simulink model "complete_fusion_syste"  (R2022b)
settings: Solver=VariableStepAuto  StartTime=0.0  StopTime=45  FixedStep=t  RelTol=1e-3
values from neighbouring files (symbols this model uses):
  covA = 610    [fusion.m]    (also in fusion_parameters.m = 800; fusion_test.m = 0.00171675)
  covG = 0.76e-5    (= 7.6e-06)    [fusion.m]    (also in fusion_parameters.m = 0.0001; fusion_test.m = 0.004)
  covM = 0.4    [fusion.m]    (also in fusion_parameters.m = 80; fusion_test.m = 0)
  covP = 4    [fusion.m]    (also in fusion_parameters.m = 34; fusion_test.m = 0)
  covV = 0.01    [fusion.m]    (also in fusion_parameters.m = 0.0464; fusion_test.m = 0)
  fusion_t = 0.005    [fusion_parameters.m]
  gps_hz = 1/25    (= 0.04)    [fusion_parameters.m]
  imu_hz = 0.015    [fusion_parameters.m]
  IMUNED2VNED = rotmat(quaternion(IMU_ANGLE,"eulerd","XYZ","frame"),"frame")    [fusion_parameters.m]
  initstate = zeros(28,1)    [fusion_parameters.m]    (also in fusion_test.m)
  MAGNED2VNED = rotmat(quaternion(MAG_ANGLE,"eulerd","XYZ","frame"),"frame")    [fusion_parameters.m]
  ref_location = [40.437675, -86.943750, 680]    [fusion_parameters.m]
libraries: simulink x2, sensorgpslib x1, mspsensorlib x1
settings Model: Creator=fullb  LastModifiedBy=Inver

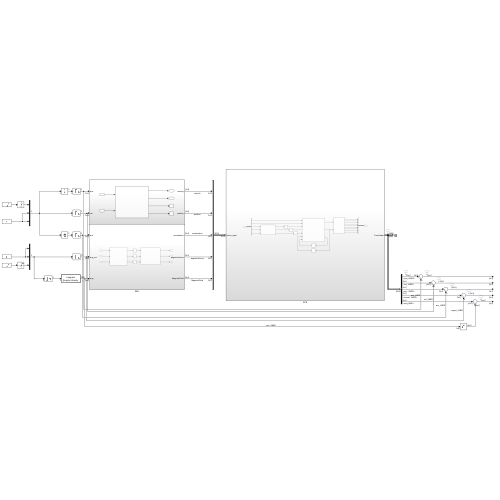
[thumbnail: Simulink's stored preview of the top-level diagram]
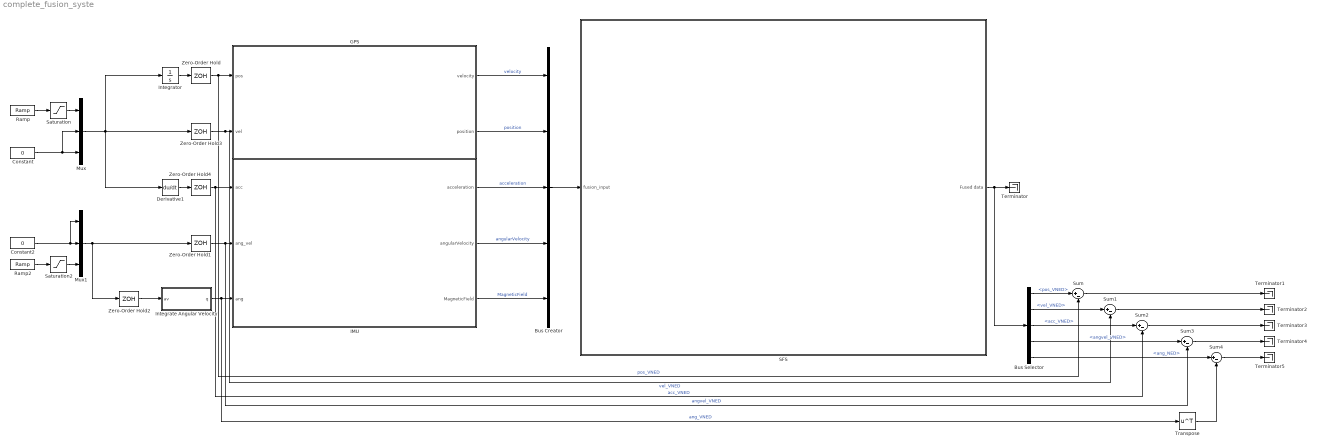
== system complete_fusion_syste ==
  Bus Creator : BusCreator  Inputs=5
  Bus Selector : BusSelector  OutputSignals=pos_VNED,vel_VNED,acc_VNED,angvel_VNED,ang_NED
  Constant : Constant  Value=0
  Constant2 : Constant  Value=0
  Derivative1 : Derivative
  GPS : Subsystem
  IMU : Subsystem
  Integrate Angular Velocity : MATLAB Function  TreatAsAtomicUnit=on  mask{rate=imu_hz}
      mask prompts: rate "Sample Rate"
  Integrator : Integrator
  Mux : Mux  Inputs=3
  Mux1 : Mux  Inputs=3
  Ramp : simulink/Sources/Ramp  slope=3  start=0  InitialOutput=-30
  Ramp2 : simulink/Sources/Ramp  slope=1  start=0  InitialOutput=-20
  SFS : Subsystem
  Saturation : Saturate  UpperLimit=10  LowerLimit=0
  Saturation2 : Saturate  UpperLimit=2  LowerLimit=0
  Sum{,1..4} (5 alike) : Sum  Inputs=|+-
  Terminator{,1..5} (6 alike) : Terminator
  Transpose : Math  Operator=transpose
  Zero-Order Hold : ZeroOrderHold  SampleTime=gps_hz
  Zero-Order Hold1 : ZeroOrderHold  SampleTime=imu_hz
  Zero-Order Hold2 : ZeroOrderHold  SampleTime=imu_hz
  Zero-Order Hold3 : ZeroOrderHold  SampleTime=gps_hz
  Zero-Order Hold4 : ZeroOrderHold  SampleTime=imu_hz
  wires:
  Bus Creator/1 -> SFS/1(fusion_input)
  SFS/1(Fused data) -> Bus Selector/1, Terminator/1
  GPS/1(velocity) -> Bus Creator/1  "velocity"
  GPS/2(position) -> Bus Creator/2  "position"
  IMU/1(acceleration) -> Bus Creator/3  "acceleration"
  IMU/2(angularVelocity) -> Bus Creator/4  "angularVelocity"
  IMU/3(MagneticField) -> Bus Creator/5  "MagneticField"
  Mux/1 -> Zero-Order Hold3/1, Derivative1/1, Integrator/1
  Derivative1/1 -> Zero-Order Hold4/1
  Ramp/1 -> Saturation/1
  Constant/1 -> Mux/2, Mux/3
  Zero-Order Hold1/1 -> Sum3/2, IMU/2(ang_vel)  "angvel_VNED"
  Zero-Order Hold2/1 -> Integrate Angular Velocity/1(av)
  Zero-Order Hold/1 -> Sum/2, GPS/1(pos)  "pos_VNED"
  Zero-Order Hold3/1 -> Sum1/2, GPS/2(vel)  "vel_VNED"
  Zero-Order Hold4/1 -> Sum2/2, IMU/1(acc)  "acc_VNED"
  Integrator/1 -> Zero-Order Hold/1
  Saturation/1 -> Mux/1
  Constant2/1 -> Mux1/1, Mux1/2
  Saturation2/1 -> Mux1/3
  Ramp2/1 -> Saturation2/1
  Mux1/1 -> Zero-Order Hold2/1, Zero-Order Hold1/1
  Integrate Angular Velocity/1(q) -> Transpose/1, IMU/3(ang)  "ang_VNED"
  Bus Selector/1 -> Sum/1  "<pos_VNED>"
  Bus Selector/2 -> Sum1/1  "<vel_VNED>"
  Bus Selector/3 -> Sum2/1  "<acc_VNED>"
  Bus Selector/4 -> Sum3/1  "<angvel_VNED>"
  Bus Selector/5 -> Sum4/1  "<ang_NED>"
  Sum/1 -> Terminator1/1
  Sum1/1 -> Terminator2/1
  Sum2/1 -> Terminator3/1
  Sum3/1 -> Terminator4/1
  Sum4/1 -> Terminator5/1
  Transpose/1 -> Sum4/2

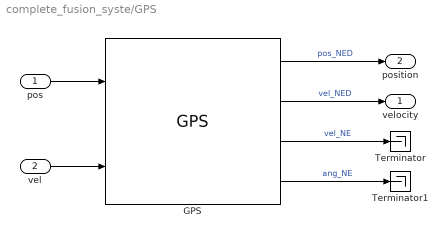
== system complete_fusion_syste/GPS ==
  pos : Inport  PortDimensions=[1 3]
  vel : Inport  Port=2  PortDimensions=[1 3]
  GPS : sensorgpslib/GPS  DispRefFrame=NED  PositionInputFormat=Local  ReferenceLocation=ref_location  HorizontalPositionAccuracy=GPS_Z_ACCURACY  VerticalPositionAccuracy=GPS_XY_ACCURACY  VelocityAccuracy=GPS_V_ACCURACY  DecayFactor=GPS_NOISE_FACTOR  SeedDouble=r_GPS  SimulateUsing=Interpreted execution
      settings: LibrarySourceBlock=mspsensorlib/GPS
  Terminator : Terminator
  Terminator1 : Terminator
  velocity : Outport
  position : Outport  Port=2
  wires:
  GPS/1 -> position/1  "pos_NED"
  GPS/2 -> velocity/1  "vel_NED"
  GPS/3 -> Terminator/1  "vel_NE"
  GPS/4 -> Terminator1/1  "ang_NE"
  pos/1 -> GPS/1
  vel/1 -> GPS/2

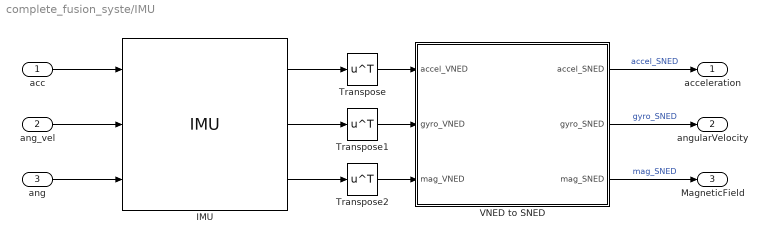
== system complete_fusion_syste/IMU ==
  acc : Inport  PortDimensions=[1 3]
  ang_vel : Inport  Port=2  PortDimensions=[1 3]
  ang : Inport  Port=3  PortDimensions=[1 4]
  IMU : mspsensorlib/IMU  DispRefFrame=NED  Temperature=25  MagneticFieldNED=ref_mag_field  MagneticFieldENU=[ -2.4169, 27.5550, 16.0849 ]  SeedDouble=r_IMU  SimulateUsing=Interpreted execution  AccelParamsMeasurementRange=ACC_MAX  AccelParamsResolution=ACC_RES  AccelParamsConstantBias=ACC_BIAS  AccelParamsAxesMisalignment=ACC_SKEW  AccelParamsNoiseDensity=ACC_VEL_WALK  AccelParamsBiasInstability=ACC_BIAS_INSTABILITY  AccelParamsRandomWalk=ACC_WALK  AccelParamsTemperatureBias=ACC_T_BIAS  AccelParamsTemperatureScaleFactor=ACC_T_SCALE  GyroParamsMeasurementRange=GYR_MAX  GyroParamsResolution=GYR_RES  GyroParamsConstantBias=GYR_BIAS  GyroParamsAxesMisalignment=GYR_SKEW  GyroParamsAccelerationBias=GYR_ACC_BIAS  GyroParamsNoiseDensity=GYR_ANG_WALK  GyroParamsBiasInstability=GYR_BIAS_INSTABILITY  GyroParamsRandomWalk=GYR_WALK  GyroParamsTemperatureBias=GYR_T_BIAS  GyroParamsTemperatureScaleFactor=GYR_T_SCALE  MagParamsMeasurementRange=MAG_MAX  MagParamsResolution=MAG_RES  MagParamsConstantBias=MAG_BIAS  MagParamsAxesMisalignment=MAG_SKEW  MagParamsNoiseDensity=MAG_WHITE  MagParamsBiasInstability=MAG_BIAS_INSTABILITY  MagParamsRandomWalk=MAG_WALK  MagParamsTemperatureBias=MAG_T_BIAS  MagParamsTemperatureScaleFactor=MAG_T_SCALE
  Transpose : Math  Operator=transpose
  Transpose1 : Math  Operator=transpose
  Transpose2 : Math  Operator=transpose
  VNED to SNED : MATLAB Function  TreatAsAtomicUnit=on
  acceleration : Outport
  angularVelocity : Outport  Port=2
  MagneticField : Outport  Port=3
  wires:
  IMU/1 -> Transpose/1
  IMU/2 -> Transpose1/1
  IMU/3 -> Transpose2/1
  ang_vel/1 -> IMU/2
  ang/1 -> IMU/3
  acc/1 -> IMU/1
  VNED to SNED/3(mag_SNED) -> MagneticField/1  "mag_SNED"
  VNED to SNED/2(gyro_SNED) -> angularVelocity/1  "gyro_SNED"
  VNED to SNED/1(accel_SNED) -> acceleration/1  "accel_SNED"
  Transpose/1 -> VNED to SNED/1(accel_VNED)
  Transpose1/1 -> VNED to SNED/2(gyro_VNED)
  Transpose2/1 -> VNED to SNED/3(mag_VNED)

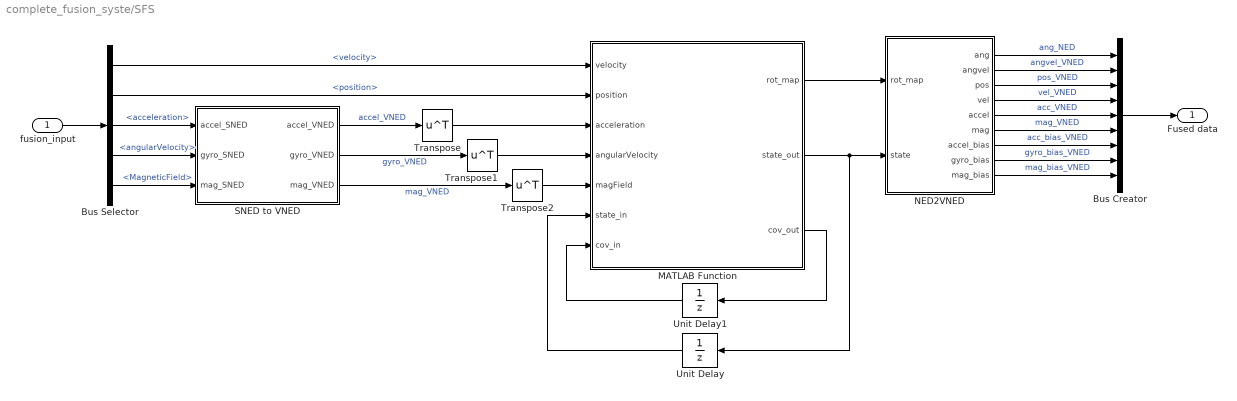
== system complete_fusion_syste/SFS ==
  fusion_input : Inport
  Bus Creator : BusCreator  Inputs=9
  Bus Selector : BusSelector  OutputSignals=velocity,position,acceleration,angularVelocity,MagneticField
  MATLAB Function : MATLAB Function  TreatAsAtomicUnit=on  SystemSampleTime=fusion_t
  NED2VNED : MATLAB Function  TreatAsAtomicUnit=on
  SNED to VNED : MATLAB Function  TreatAsAtomicUnit=on  SystemSampleTime=fusion_t
  Transpose : Math  Operator=transpose
  Transpose1 : Math  Operator=transpose
  Transpose2 : Math  Operator=transpose
  Unit Delay : UnitDelay  InitialCondition=initstate  SampleTime=fusion_t  HasFrameUpgradeWarning=on
  Unit Delay1 : UnitDelay  InitialCondition=eye(28)./1000  SampleTime=fusion_t  HasFrameUpgradeWarning=on
  Fused data : Outport
  wires:
  Bus Selector/1 -> MATLAB Function/1(velocity)  "<velocity>"
  Bus Selector/4 -> SNED to VNED/2(gyro_SNED)  "<angularVelocity>"
  Unit Delay/1 -> MATLAB Function/6(state_in)
  MATLAB Function/2(state_out) -> Unit Delay/1, NED2VNED/2(state)
  Bus Selector/2 -> MATLAB Function/2(position)  "<position>"
  Bus Selector/3 -> SNED to VNED/1(accel_SNED)  "<acceleration>"
  fusion_input/1 -> Bus Selector/1
  Bus Selector/5 -> SNED to VNED/3(mag_SNED)  "<MagneticField>"
  MATLAB Function/1(rot_map) -> NED2VNED/1(rot_map)
  Bus Creator/1 -> Fused data/1
  SNED to VNED/2(gyro_VNED) -> Transpose1/1  "gyro_VNED"
  SNED to VNED/1(accel_VNED) -> Transpose/1  "accel_VNED"
  SNED to VNED/3(mag_VNED) -> Transpose2/1  "mag_VNED"
  MATLAB Function/3(cov_out) -> Unit Delay1/1
  Unit Delay1/1 -> MATLAB Function/7(cov_in)
  NED2VNED/1(ang) -> Bus Creator/1  "ang_NED"
  NED2VNED/2(angvel) -> Bus Creator/2  "angvel_VNED"
  NED2VNED/6(mag) -> Bus Creator/6  "mag_VNED"
  NED2VNED/3(pos) -> Bus Creator/3  "pos_VNED"
  NED2VNED/4(vel) -> Bus Creator/4  "vel_VNED"
  NED2VNED/5(accel) -> Bus Creator/5  "acc_VNED"
  NED2VNED/7(accel_bias) -> Bus Creator/7  "acc_bias_VNED"
  NED2VNED/8(gyro_bias) -> Bus Creator/8  "gyro_bias_VNED"
  NED2VNED/9(mag_bias) -> Bus Creator/9  "mag_bias_VNED"
  Transpose/1 -> MATLAB Function/3(acceleration)
  Transpose1/1 -> MATLAB Function/4(angularVelocity)
  Transpose2/1 -> MATLAB Function/5(magField)

== matlab function complete_fusion_syste/SFS/SNED to VNED ==
  data: accel_VNED output size=[3 1]; gyro_VNED output size=[3 1]; accel_SNED input; gyro_SNED input; mag_SNED input; mag_VNED output size=[3 1]; IMUNED2VNED parameter; MAGNED2VNED parameter
function [accel_VNED, gyro_VNED, mag_VNED] = SNED2VNED(accel_SNED, gyro_SNED, mag_SNED, IMUNED2VNED, MAGNED2VNED)
%% Coordinate Transformation
accel_VNED = IMUNED2VNED*accel_SNED;
gyro_VNED = IMUNED2VNED*gyro_SNED;
mag_VNED = MAGNED2VNED*mag_SNED;

end

== matlab function complete_fusion_syste/Integrate Angular Velocity ==
  data: av input; q output; rate parameter
function q = integrateAngVel(av, rate)
%INTEGRATEANGVEL Integrate angular velocity to a quaternion
%  Treat Angular Velocity as an incremental rotation vector.

%   Copyright 2019 The MathWorks, Inc.   

persistent orient
if isempty(orient)
    % Initial orientation is the identity quaternion.
    orient = cast(quaternion(1,0,0,0), 'like', av);
end

% Convert angular velocity to a rotation vector.
rv = quaternion(av'*(rate), 'rotvec');
orient = rv * orient;
q = compact(orient);

== matlab function complete_fusion_syste/SFS/MATLAB Function ==
  data: rot_map output; velocity input size=[1,3]; state_out output; position input size=[1,3]; acceleration input size=[1,3]; angularVelocity input size=[1,3]; magField input size=[1,3]; state_in input; cov_in input; covG parameter; covA parameter; covM parameter; covP parameter; covV parameter; fusion_t parameter; ref_location parameter; cov_out output
function [rot_map, state_out, cov_out] = fusion(velocity, position ,acceleration,angularVelocity, magField, state_in, cov_in, covG, covA, covM, covP, covV, fusion_t, ref_location) 

% creating the filter and loading previous state 
filter = insfilterAsync();
filter.ReferenceLocation = ref_location;
filter.State = state_in;
filter.StateCovariance = cov_in;

filter.AccelerationNoise = [1 1 1].*5;

% update filter state
predict(filter, fusion_t);

% Enforce Planar Conditions
position(3) = filter.ReferenceLocation(3);
velocity(3) = 0;

% the actual fusion
fuseaccel(filter,acceleration,covA);
fusegyro(filter,angularVelocity,covG);
fusemag(filter, magField,covM);
fusegps(filter,position,covP,velocity,covV);

[~,rot_map,~] = pose(filter, 'rotmat');

% Output matricies
state_out = filter.State;
cov_out = filter.StateCovariance;

end

== matlab function complete_fusion_syste/SFS/NED2VNED ==
  data: rot_map input; state input; ang output; angvel output; pos output; vel output; accel output; mag output; accel_bias output; gyro_bias output; mag_bias output
function [ang,angvel,pos,vel,accel,mag,accel_bias,gyro_bias,mag_bias] = NED2VNED(rot_map,state)

ang = state(1:4);                    % quaternion (VNED2SNED)
angvel = state(5:7);                 % chassis angular velocity (rad/s)(VNED)
pos = rot_map*state(8:10);           % chassis position (m)(VNED)
vel = rot_map*state(11:13);          % chassis velocity (m/s)(VNED)
accel = rot_map*state(14:16);        % chassis acceleration (m/s^2)(VNED)
mag = rot_map*state(23:25);          % magnetic field (uT)(VNED)

accel_bias = rot_map*state(17:19);   % accelerometer bias (m/s^2)(VNED)
gyro_bias = rot_map*state(20:22);    % gyroscope bias (rad/s)(VNED)
mag_bias = rot_map*state(26:28);     % magnetometer bias (uT)(VNED)

end

== matlab function complete_fusion_syste/IMU/VNED to SNED ==
  data: accel_SNED output; gyro_SNED output; accel_VNED input size=[3 1]; gyro_VNED input size=[3 1]; mag_VNED input size=[3 1]; mag_SNED output; IMUNED2VNED parameter; MAGNED2VNED parameter
function [accel_SNED, gyro_SNED, mag_SNED] = VNED2SNED(accel_VNED, gyro_VNED, mag_VNED, IMUNED2VNED, MAGNED2VNED)
%% Coordinate Transformation
accel_SNED = IMUNED2VNED\accel_VNED;
gyro_SNED = IMUNED2VNED\gyro_VNED;
mag_SNED = MAGNED2VNED\mag_VNED;

end
